simulink model "Copy_of_EMB_LRM_LaneRoleManager"  (R2025a)
settings: Solver=FixedStepDiscrete  StartTime=0.0  StopTime=inf  FixedStep=0.01  RelTol=1e-3
(part 2 of 2)

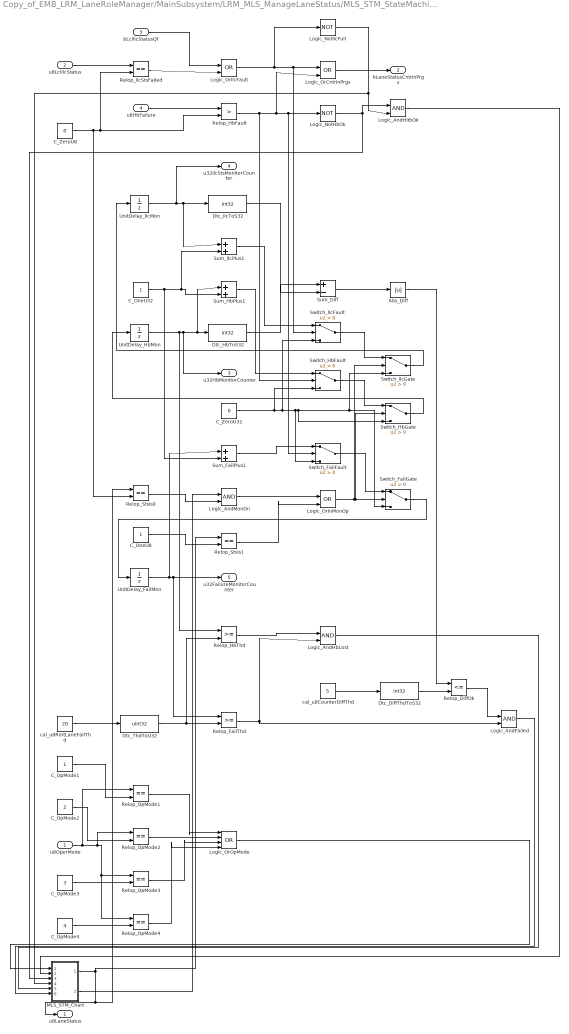
== system Copy_of_EMB_LRM_LaneRoleManager/MainSubsystem/LRM_MLS_ManageLaneStatus/MLS_STM_StateMachine ==
  u8OperMode : Inport  Description=系统运行模式；类型 uint8；范围 0..5  OutDataTypeStr=uint8
  u8LclIlcStatus : Inport  Description=本控制链路 ILC 状态；类型 uint8；范围 0..2  Port=2  OutDataTypeStr=uint8
  bLclIlcStatusQf : Inport  Description=本控制链路 ILC 状态信号质量（1=异常）；类型 boolean  Port=3  OutDataTypeStr=boolean
  u8HbFailure : Inport  Description=心跳丢失故障判断（来自 MLS_HB_Failure）；类型 uint8；范围 0..1  Port=4  OutDataTypeStr=uint8
  Abs_Diff : Abs  Description=计数器差值绝对值  SaturateOnIntegerOverflow=off
  C_OneU32 : Constant  Description=计数器步长 1；uint32  OutDataTypeStr=uint32
  C_OneU8 : Constant  Description=常量 1（LANE_STS_OPERATING=1）；uint8  OutDataTypeStr=uint8
  C_OpMode1 : Constant  Description=OPMODE_NORMAL_OPERATION=1；uint8  OutDataTypeStr=uint8
  C_OpMode2 : Constant  Description=OPMODE_LIMP_HOME=2；uint8  Value=2  OutDataTypeStr=uint8
  C_OpMode3 : Constant  Description=OPMODE_LIMP_ASIDE=3；uint8  Value=3  OutDataTypeStr=uint8
  C_OpMode4 : Constant  Description=OPMODE_CRAWL=4；uint8  Value=4  OutDataTypeStr=uint8
  C_ZeroU32 : Constant  Description=计数器清零常量；uint32  Value=0  OutDataTypeStr=uint32
  C_ZeroU8 : Constant  Description=零常量；uint8  Value=0  OutDataTypeStr=uint8
  Dtc_DiffThdToS32 : DataTypeConversion  Description=差值阈值转 int32  OutDataTypeStr=int32  SaturateOnIntegerOverflow=off  RndMeth=Floor
  Dtc_HbToS32 : DataTypeConversion  Description=Hb 计数器转 int32  OutDataTypeStr=int32  SaturateOnIntegerOverflow=off  RndMeth=Floor
  Dtc_IlcToS32 : DataTypeConversion  Description=ILC 计数器转 int32  OutDataTypeStr=int32  SaturateOnIntegerOverflow=off  RndMeth=Floor
  Dtc_ThdToU32 : DataTypeConversion  Description=窗口阈值转 uint32 供计数器比较  OutDataTypeStr=uint32  SaturateOnIntegerOverflow=off  RndMeth=Floor
  Logic_AndFailed : Logic  Description=Failed 进入条件  IconShape=distinctive  AllPortsSameDT=off  OutDataTypeStr=boolean
  Logic_AndHbLost : Logic  Description=HbLost 进入条件  IconShape=distinctive  AllPortsSameDT=off  OutDataTypeStr=boolean
  Logic_AndHlthOk : Logic  Description=健康条件：心跳正常且 ILC 正常  IconShape=distinctive  AllPortsSameDT=off  OutDataTypeStr=boolean
  Logic_AndMonOn : Logic  Description=INIT.MonitoringOn 状态  IconShape=distinctive  AllPortsSameDT=off  OutDataTypeStr=boolean
  Logic_NotHbOk : Logic  Description=心跳正常  Operator=NOT  Inputs=1  IconShape=distinctive  AllPortsSameDT=off  OutDataTypeStr=boolean
  Logic_NotIlcFull : Logic  Description=ILC 正常（质量好且状态非 Failed）  Operator=NOT  Inputs=1  IconShape=distinctive  AllPortsSameDT=off  OutDataTypeStr=boolean
  Logic_OrCntrInPrgs : Logic  Description=LaneStatusCntrInPrgs：心跳故障或 ILC 异常  Operator=OR  IconShape=distinctive  AllPortsSameDT=off  OutDataTypeStr=boolean
  Logic_OrIlcFault : Logic  Description=ILC 异常：质量异常(1) 或 状态==Failed  Operator=OR  IconShape=distinctive  AllPortsSameDT=off  OutDataTypeStr=boolean
  Logic_OrInMonOp : Logic  Description=监控计数激活状态：MonitoringOn 或 Operating  Operator=OR  IconShape=distinctive  AllPortsSameDT=off  OutDataTypeStr=boolean
  Logic_OrOpMode : Logic  Description=监控激活条件：运行模式属于 {NORMAL,LIMP_HOME,LIMP_ASIDE,CRAWL}  Operator=OR  Inputs=4  IconShape=distinctive  AllPortsSameDT=off  OutDataTypeStr=boolean
  MLS_STM_Chart : Stateflow chart  Description=MLS_STM_StateMachine 布尔门控 Stateflow：输入全为 boolean 条件，输出 u8LaneStatus(0..3) 与 bMonActive；状态 INIT.MonitoringOff/On、Operating、HbLost、Failed，优先级 Operating>Failed>HbLost  TreatAsAtomicUnit=on
  Relop_DiffOk : RelationalOperator  Description=abs(Hb-ILC) <= 差值阈值  Operator=<=  OutDataTypeStr=boolean  RndMeth=Simplest  InputSameDT=off
  Relop_FailThd : RelationalOperator  Description=故障计数器 >= 窗口阈值  OutDataTypeStr=boolean  RndMeth=Simplest  InputSameDT=off
  Relop_HbFault : RelationalOperator  Description=心跳故障：u8HbFailure > 0  Operator=>  OutDataTypeStr=boolean  RndMeth=Simplest  InputSameDT=off
  Relop_HbThd : RelationalOperator  Description=Hb 计数器 >= 窗口阈值  OutDataTypeStr=boolean  RndMeth=Simplest  InputSameDT=off
  Relop_IlcStsFailed : RelationalOperator  Description=ILC 状态==Failed  Operator===  OutDataTypeStr=boolean  RndMeth=Simplest  InputSameDT=off
  Relop_OpMode1 : RelationalOperator  Description=运行模式==NORMAL_OPERATION  Operator===  OutDataTypeStr=boolean  RndMeth=Simplest  InputSameDT=off
  Relop_OpMode2 : RelationalOperator  Description=运行模式==LIMP_HOME  Operator===  OutDataTypeStr=boolean  RndMeth=Simplest  InputSameDT=off
  Relop_OpMode3 : RelationalOperator  Description=运行模式==LIMP_ASIDE  Operator===  OutDataTypeStr=boolean  RndMeth=Simplest  InputSameDT=off
  Relop_OpMode4 : RelationalOperator  Description=运行模式==CRAWL  Operator===  OutDataTypeStr=boolean  RndMeth=Simplest  InputSameDT=off
  Relop_StsIs0 : RelationalOperator  Description=LaneStatus==INITIALISING(0)  Operator===  OutDataTypeStr=boolean  RndMeth=Simplest  InputSameDT=off
  Relop_StsIs1 : RelationalOperator  Description=LaneStatus==OPERATING(1)  Operator===  OutDataTypeStr=boolean  RndMeth=Simplest  InputSameDT=off
  Sum_Diff : Sum  Description=Hb-ILC 差值  Inputs=+-
  Sum_FailPlus1 : Sum  Description=故障计数器 +1  Inputs=|++
  Sum_HbPlus1 : Sum  Description=Hb 计数器 +1  Inputs=|++
  Sum_IlcPlus1 : Sum  Description=ILC 计数器 +1  Inputs=|++
  Switch_FailFault : Switch  Description=心跳故障时计数+1，否则清零  Criteria=u2 > Threshold  SaturateOnIntegerOverflow=off  InputSameDT=off
  Switch_FailGate : Switch  Description=监控激活时保持计数，否则清零  Criteria=u2 > Threshold  SaturateOnIntegerOverflow=off  InputSameDT=off
  Switch_HbFault : Switch  Description=Hb 故障时计数+1，否则清零  Criteria=u2 > Threshold  SaturateOnIntegerOverflow=off  InputSameDT=off
  Switch_HbGate : Switch  Description=监控激活时保持计数，否则清零  Criteria=u2 > Threshold  SaturateOnIntegerOverflow=off  InputSameDT=off
  Switch_IlcFault : Switch  Description=ILC 故障时计数+1，否则清零  Criteria=u2 > Threshold  SaturateOnIntegerOverflow=off  InputSameDT=off
  Switch_IlcGate : Switch  Description=监控激活时保持计数，否则清零  Criteria=u2 > Threshold  SaturateOnIntegerOverflow=off  InputSameDT=off
  UnitDelay_FailMon : UnitDelay  Description=故障监控计数器状态；uint32  SampleTime=-1  HasFrameUpgradeWarning=on
  UnitDelay_HbMon : UnitDelay  Description=Hb 监控计数器状态；uint32  SampleTime=-1  HasFrameUpgradeWarning=on
  UnitDelay_IlcMon : UnitDelay  Description=ILC 监控计数器状态；uint32  SampleTime=-1  HasFrameUpgradeWarning=on
  cal_u8CounterDiffThd : Constant  Description=cal_u8CounterDiffThd；Hb 与 ILC 监控计数器差值阈值；uint8；1..255；默认 5  Value=5  OutDataTypeStr=uint8
  cal_u8RmtLaneFallThd : Constant  Description=cal_u8RmtLaneFallThd；故障监控窗口阈值（周期数）；uint8；1..255；默认 20  Value=20  OutDataTypeStr=uint8
  u8LaneStatus : Outport  Description=控制链路健康状态；类型 uint8；范围 0..3
  bLaneStatusCntrInPrgs : Outport  Description=状态切换计数器进行中标志；类型 boolean  Port=2
  u32HbMonitorCounter : Outport  Description=心跳监控计数器；类型 uint32  Port=3
  u32IlcStsMonitorCounter : Outport  Description=ILC 状态监控计数器；类型 uint32  Port=4
  u32FailureMonitorCounter : Outport  Description=故障监控计数器；类型 uint32  Port=5
  wires:
  Relop_DiffOk/1 -> Logic_AndFailed/1
  Dtc_DiffThdToS32/1 -> Relop_DiffOk/2
  cal_u8CounterDiffThd/1 -> Dtc_DiffThdToS32/1
  Abs_Diff/1 -> Relop_DiffOk/1
  Sum_Diff/1 -> Abs_Diff/1
  Dtc_IlcToS32/1 -> Sum_Diff/2
  Dtc_HbToS32/1 -> Sum_Diff/1
  Relop_FailThd/1 -> Logic_AndHbLost/2, Logic_AndFailed/2
  Relop_HbThd/1 -> Logic_AndHbLost/1
  Dtc_ThdToU32/1 -> Relop_HbThd/2, Relop_FailThd/2
  cal_u8RmtLaneFallThd/1 -> Dtc_ThdToU32/1
  Switch_FailGate/1 -> UnitDelay_FailMon/1
  Switch_FailFault/1 -> Switch_FailGate/1
  Sum_FailPlus1/1 -> Switch_FailFault/1
  UnitDelay_FailMon/1 -> u32FailureMonitorCounter/1, Relop_FailThd/1, Sum_FailPlus1/1
  Switch_IlcGate/1 -> UnitDelay_IlcMon/1
  Switch_IlcFault/1 -> Switch_IlcGate/1
  Sum_IlcPlus1/1 -> Switch_IlcFault/1
  UnitDelay_IlcMon/1 -> Sum_IlcPlus1/1, Dtc_IlcToS32/1, u32IlcStsMonitorCounter/1
  Switch_HbGate/1 -> UnitDelay_HbMon/1
  Switch_HbFault/1 -> Switch_HbGate/1
  C_ZeroU32/1 -> Switch_IlcGate/3, Switch_FailGate/3, Switch_HbGate/3, Switch_FailFault/3, Switch_IlcFault/3, Switch_HbFault/3
  Sum_HbPlus1/1 -> Switch_HbFault/1
  C_OneU32/1 -> Sum_HbPlus1/2, Sum_IlcPlus1/2, Sum_FailPlus1/2
  UnitDelay_HbMon/1 -> Sum_HbPlus1/1, Dtc_HbToS32/1, u32HbMonitorCounter/1, Relop_HbThd/1
  Logic_OrInMonOp/1 -> Switch_HbGate/2, Switch_FailGate/2, Switch_IlcGate/2
  Relop_StsIs1/1 -> Logic_OrInMonOp/2
  Logic_AndMonOn/1 -> Logic_OrInMonOp/1
  C_OneU8/1 -> Relop_StsIs1/2
  Relop_StsIs0/1 -> Logic_AndMonOn/2
  Logic_OrCntrInPrgs/1 -> bLaneStatusCntrInPrgs/1
  Logic_NotIlcFull/1 -> MLS_STM_Chart/4(bIlcFull), Logic_AndHlthOk/2
  Logic_NotHbOk/1 -> Logic_AndHlthOk/1, MLS_STM_Chart/3(bHbOk)
  Relop_HbFault/1 -> Logic_NotHbOk/1, Switch_FailFault/2, Logic_OrCntrInPrgs/2, Switch_HbFault/2
  u8HbFailure/1 -> Relop_HbFault/1
  Logic_OrIlcFault/1 -> Logic_OrCntrInPrgs/1, Switch_IlcFault/2, Logic_NotIlcFull/1
  Relop_IlcStsFailed/1 -> Logic_OrIlcFault/2
  bLclIlcStatusQf/1 -> Logic_OrIlcFault/1
  C_ZeroU8/1 -> Relop_IlcStsFailed/2, Relop_HbFault/2, Relop_StsIs0/2
  u8LclIlcStatus/1 -> Relop_IlcStsFailed/1
  Relop_OpMode4/1 -> Logic_OrOpMode/4
  Relop_OpMode3/1 -> Logic_OrOpMode/3
  Relop_OpMode2/1 -> Logic_OrOpMode/2
  Relop_OpMode1/1 -> Logic_OrOpMode/1
  C_OpMode4/1 -> Relop_OpMode4/2
  C_OpMode3/1 -> Relop_OpMode3/2
  C_OpMode2/1 -> Relop_OpMode2/2
  C_OpMode1/1 -> Relop_OpMode1/2
  u8OperMode/1 -> Relop_OpMode3/1, Relop_OpMode4/1, Relop_OpMode2/1, Relop_OpMode1/1
  Logic_OrOpMode/1 -> MLS_STM_Chart/1(bMonitoringActive)
  Logic_AndHlthOk/1 -> MLS_STM_Chart/2(bHlthOk)
  Logic_AndHbLost/1 -> MLS_STM_Chart/5(bHbLostCond)
  Logic_AndFailed/1 -> MLS_STM_Chart/6(bFailedCond)
  MLS_STM_Chart/1(u8LaneStatus) -> u8LaneStatus/1, Relop_StsIs0/1, Relop_StsIs1/1
  MLS_STM_Chart/2(bMonActive) -> Logic_AndMonOn/1

== stateflow chart Copy_of_EMB_LRM_LaneRoleManager/MainSubsystem/LRM_MLR_ManageLaneRole/MLR_STM_Chart ==
  state MLR_STM_OperationalRoles
    state MLR_STM_FallBack
      en: u8LaneRole = uint8(3);
    state MLR_STM_Support
      en: u8LaneRole = uint8(4);
    state MLR_STM_Master
      en: u8LaneRole = uint8(2);
    (default) -> MLR_STM_FallBack
    MLR_STM_FallBack -> MLR_STM_Master [order 1] : [bFallback2Master]
    MLR_STM_Master -> MLR_STM_FallBack [order 2] : [bMaster2Fallback]
    MLR_STM_FallBack -> MLR_STM_Support [order 3] : [bFallback2Support]
    MLR_STM_FallBack -> MLR_STM_Support [order 4] : [bFallback2SupportUnknown]
    MLR_STM_Support -> MLR_STM_FallBack [order 3] : [bSupport2Fallback]
    MLR_STM_FallBack -> MLR_STM_Master [order 2] : [bFallback2MasterTakeover]
    MLR_STM_Master -> MLR_STM_FallBack [order 3] : [bMaster2FallbackImmediate]
    MLR_STM_Support -> MLR_STM_Master [order 2] : [bSupport2MasterTakeover]
    MLR_STM_Support -> MLR_STM_Master [order 1] : [bSupport2Master]
    MLR_STM_Master -> MLR_STM_Support [order 1] : [bMaster2Support]
  state MLR_STM_Disabled
    en: u8LaneRole = uint8(5);
  state MLR_STM_Init
    en: u8LaneRole = uint8(1);
  state MLR_STM_ShuttingDown
    en: u8LaneRole = uint8(6);
  MLR_STM_Init -> MLR_STM_FallBack [order 4] : [bArbRmtMaster]
  MLR_STM_Init -> MLR_STM_Master [order 3] : [bArbLclGtRmt]
  MLR_STM_OperationalRoles -> MLR_STM_Disabled [order 2] : [bLclDisabled]
  MLR_STM_OperationalRoles -> MLR_STM_ShuttingDown [order 1] : [bShutdown]
  MLR_STM_Init -> MLR_STM_Disabled [order 2] : [bLclDisabled]
  (default) -> MLR_STM_Init
  MLR_STM_Disabled -> MLR_STM_ShuttingDown : [bShutdown]
  MLR_STM_ShuttingDown -> MLR_STM_Init : [bNotShutdown]
  MLR_STM_Init -> MLR_STM_ShuttingDown [order 1] : [bShutdown]
  data: bShutdown input boolean; bNotShutdown input boolean; bLclDisabled input boolean; bArbLclGtRmt input boolean; bArbRmtMaster input boolean; bMaster2Support input boolean; bMaster2Fallback input boolean; bMaster2FallbackImmediate input boolean; bFallback2Master input boolean; bFallback2MasterTakeover input boolean; bFallback2Support input boolean; bFallback2SupportUnknown input boolean; bSupport2Master input boolean; bSupport2MasterTakeover input boolean; bSupport2Fallback input boolean; u8LaneRole output uint8

== stateflow chart Copy_of_EMB_LRM_LaneRoleManager/MainSubsystem/LRM_MLS_ManageLaneStatus/MLS_STM_StateMachine/MLS_STM_Chart ==
  state INIT
    state MonitoringOff
      en: u8LaneStatus = uint8(0);
      en: bMonActive = false;
    state MonitoringOn
      en: u8LaneStatus = uint8(0);
      en: bMonActive = true;
    (default) -> MonitoringOff
    MonitoringOff -> MonitoringOn : [bMonitoringActive]
  state Operating
    en: u8LaneStatus = uint8(1);
    en: bMonActive = true;
  state HbLost
    en: u8LaneStatus = uint8(2);
    en: bMonActive = false;
  state Failed
    en: u8LaneStatus = uint8(3);
    en: bMonActive = false;
  (default) -> INIT
  MonitoringOn -> Failed [order 2] : [bFailedCond]
  MonitoringOn -> Operating [order 1] : [bHlthOk]
  MonitoringOn -> HbLost [order 3] : [bHbLostCond]
  HbLost -> Operating : [bHbOk]
  Operating -> HbLost [order 2] : [bHbLostCond]
  Failed -> Operating [order 1] : [bHbOk]
  Operating -> Failed [order 1] : [bFailedCond]
  Failed -> HbLost [order 2] : [bIlcFull]
  data: bMonitoringActive input boolean; bHlthOk input boolean; bHbOk input boolean; bIlcFull input boolean; bHbLostCond input boolean; bFailedCond input boolean; u8LaneStatus output uint8; bMonActive output boolean
